simulink model "Test_Model"  (R2022b)
settings: Solver=ode23t  StartTime=0.0  StopTime=20  RelTol=1e-3
values from neighbouring files (symbols this model uses):
  csi = 1/sqrt(2)    [Main_Script.m]
  wn = 100    [Main_Script.m]
undefined symbols (not defined in the file or in its folder): AS5600, motor
libraries: simulink_extras x3, spsTriangleGeneratorLib x1, dspsigops x1
settings Model: Creator=gotta  LastModifiedBy=gotta
settings SolverCC: ZeroCrossAlgorithm=Adaptive
settings DebuggingCC: IgnoredZcDiagnostic=none

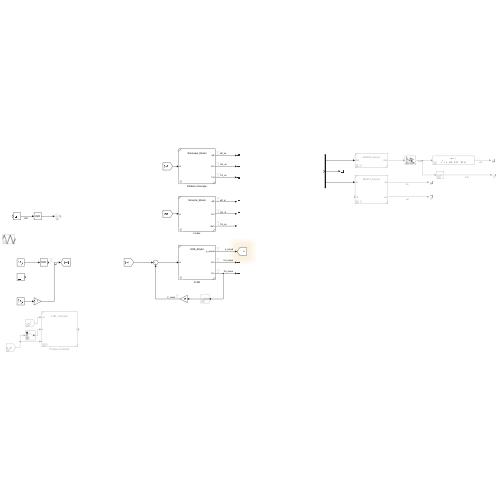
[thumbnail: Simulink's stored preview of the top-level diagram]
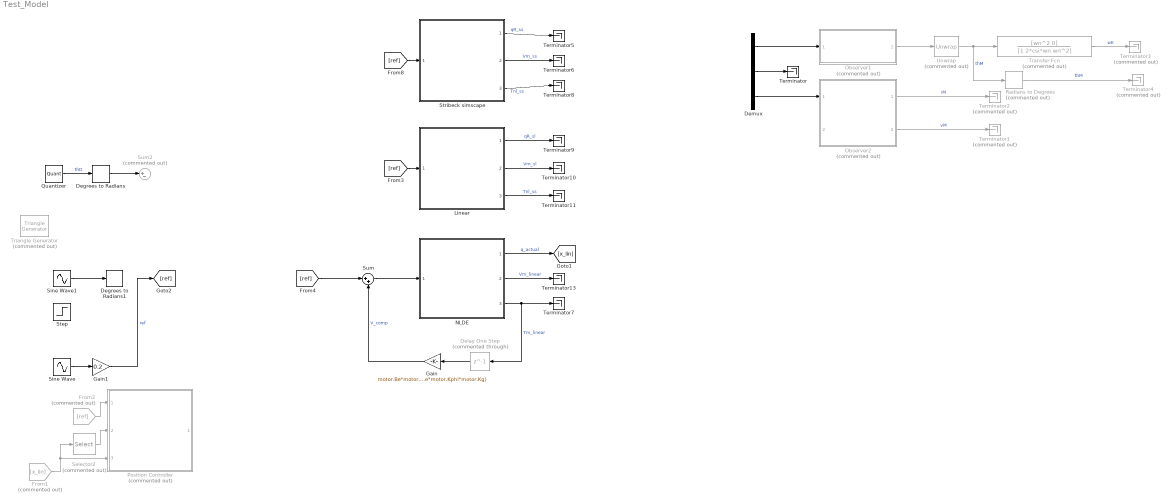
== system Test_Model ==
  Degrees to Radians : simulink_extras/Transformations/Degrees to Radians
  Degrees to Radians1 : simulink_extras/Transformations/Degrees to Radians
  Delay One Step : Delay  Commented=through  DelayLength=1  SampleTime=1e-3
  Demux : Demux  Outputs=3
  From1 : From  Commented=on  GotoTag=x_lin
  From2 : From  Commented=on  GotoTag=ref
  Gain : Gain  Gain=motor.Be*motor.La/(motor.Vcc*motor.Je*motor.Kphi*motor.Kg)
  Gain1 : Gain  Gain=0.2
  Linear : Subsystem  ReferencedSubsystem=Simulink_Model  pwr=motor.Vcc  Ra=motor.Ra  La=motor.La  Kphi=motor.Kphi  Be=motor.Be  Je=motor.Je  Kg=motor.Kg  enable_Tc=off  tau_c=motor.tau_c  enable_Tsb=off  tau_sb=motor.tau_sb  w_sb=motor.w_sb  approximate=off  lambda=1
  NLDE : Subsystem  ReferencedSubsystem=ODE_Model  pwr=motor.Vcc  Ra=motor.Ra  La=motor.La  Kphi=motor.Kphi  Be=motor.Be  Je=motor.Je  Kg=motor.Kg  enable_Tc=off  tau_c=motor.tau_c  enable_Tsb=off  tau_sb=motor.tau_sb  w_sb=motor.w_sb  approximate=off  lambda=lambda
  Observer1 : Subsystem  Commented=on  ReferencedSubsystem=AS5600_Sensor  delta_th=AS5600.q_step  wrap=on
  Observer2 : Subsystem  Commented=on  ReferencedSubsystem=INA219_Sensor  current_LSB=INA219.I_LSB  voltage_LSB=INA219.V_LSB  noise=on  i_noise_pwr=INA219.I_PSD  v_noise_pwr=INA219.V_PSD
  Position Controller : Subsystem  Commented=on  ReferencedSubsystem=LQR_controller  Kx=ctrl_lqr.Kx  Ke=ctrl_lqr.Ke
  Quantizer : Quantizer  QuantizationInterval=rad2deg(AS5600.q_step)
  Radians to Degrees : simulink_extras/Transformations/Radians to Degrees  Commented=on
  Selector2 : Selector  Commented=on  InputPortWidth=3  IndexOptions=Index vector (dialog)  Indices=1  OutputSizes=1
  Sine Wave : Sin  SampleTime=0
  Sine Wave1 : Sin  Amplitude=180  SampleTime=0
  Step : Step  After=10  SampleTime=0
  Stribeck simscape : Subsystem  ReferencedSubsystem=Simscape_Model  Ra=motor.Ra  La=motor.La  Kphi=motor.Kphi  Je=motor.Je  Be=motor.Be  tau_c=motor.tau_c  tau_sb=motor.tau_sb  w_sb=motor.w_sb  Kg=motor.Kg  pwr=motor.Vcc
  Sum : Sum  Inputs=|++
  Sum2 : Sum  Commented=on  Inputs=|+-
  Terminator{,5..11,13} (9 alike) : Terminator
  Terminator{1..4} (4 alike) : Terminator  Commented=on
  Transfer Fcn : TransferFcn  Commented=on  Numerator=[wn^2 0]  Denominator=[1 2*csi*wn wn^2]
  Triangle Generator : spsTriangleGeneratorLib/Triangle Generator  Commented=on  Freq=0.1  Phase=90  Ts=0
  Unwrap : dspsigops/Unwrap  Commented=on  tol=pi  InputProcessing=Columns as channels (frame based)  running=off
  wires:
  Stribeck simscape/2 -> Terminator6/1  "Vm_ss"
  Stribeck simscape/1 -> Terminator5/1  "qR_ss"
  Demux/3 -> Observer2/1
  Demux/2 -> Terminator/1
  Demux/1 -> Observer1/1
  Observer1/1 -> Unwrap/1
  Observer2/1 -> Terminator2/1  "iM"
  Observer2/2 -> Terminator1/1  "vM"
  Unwrap/1 -> Transfer Fcn/1, Radians to Degrees/1  "thM"
  Transfer Fcn/1 -> Terminator3/1  "wE"
  Radians to Degrees/1 -> Terminator4/1  "thM"
  Degrees to Radians/1 -> Sum2/1
  Quantizer/1 -> Degrees to Radians/1  "thD"
  NLDE/1 -> [x_lin]  "q_actual"
  Gain1/1 -> [ref]  "ref"
  NLDE/2 -> Terminator13/1  "Vm_linear"
  Sine Wave1/1 -> Degrees to Radians1/1
  Selector2/1 -> Position Controller/2
  From1/1 -> Selector2/1, Position Controller/3
  From2/1 -> Position Controller/1
  NLDE/3 -> Delay One Step/1, Terminator7/1  "Tm_linear"
  Sine Wave/1 -> Gain1/1
  [ref] -> Sum/1
  [ref] -> Stribeck simscape/1
  Stribeck simscape/3 -> Terminator8/1  "Tnl_ss"
  Sum/1 -> NLDE/1
  Delay One Step/1 -> Gain/1
  Gain/1 -> Sum/2  "V_comp"
  Linear/3 -> Terminator11/1  "Tnl_ss"
  [ref] -> Linear/1
  Linear/1 -> Terminator9/1  "qR_sl"
  Linear/2 -> Terminator10/1  "Vm_sl"
